simulink model "ref_controller"  (R2022b)
settings: Solver=VariableStepAuto  StartTime=0.0  StopTime=100.0  RelTol=1e-5
settings Model: Creator=marne  LastModifiedBy=marne

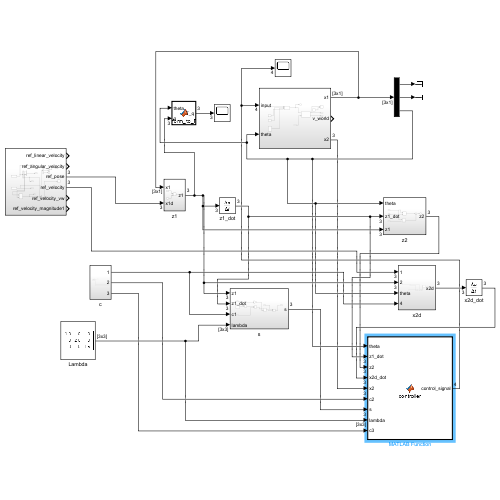
[thumbnail: Simulink's stored preview of the top-level diagram]
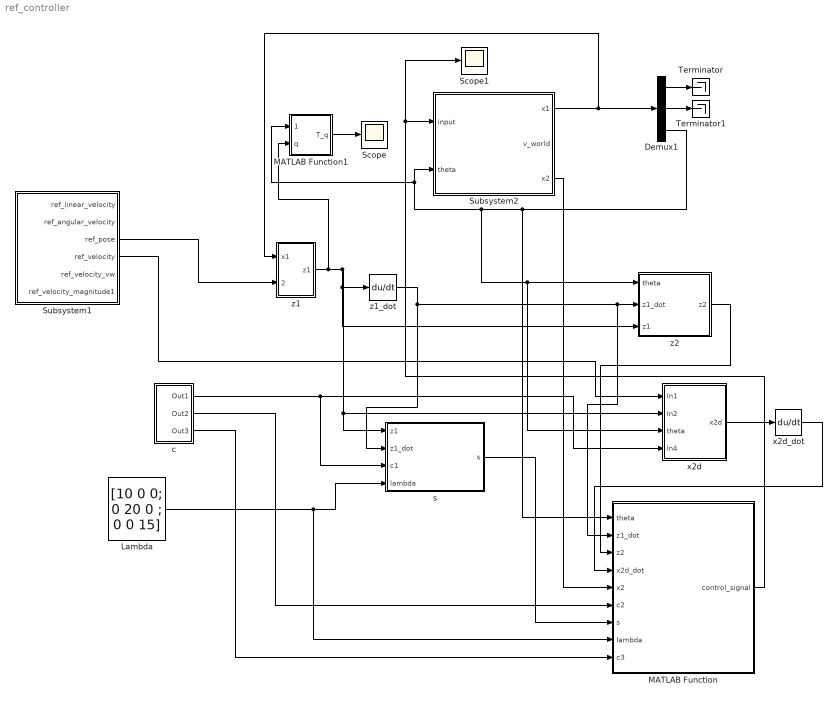
== system ref_controller ==
  Demux1 : Demux  Outputs=3
  Lambda : Constant  Value=[10 0 0; 0 20 0 ; 0 0 15]  VectorParams1D=off
  MATLAB Function : MATLAB Function  TreatAsAtomicUnit=on
  MATLAB Function1 : MATLAB Function  TreatAsAtomicUnit=on
  Scope : Scope
  Scope1 : Scope
  Subsystem1 : Subsystem
  Subsystem2 : Subsystem
  Terminator : Terminator
  Terminator1 : Terminator
  c : Subsystem
  s : Subsystem
  x2d : Subsystem
  x2d_dot : Derivative
  z1 : Subsystem
  z1_dot : Derivative
  z2 : Subsystem
  wires:
  Subsystem1/3(ref_pose) -> z1/2(x1d)
  Subsystem1/4(ref_velocity) -> x2d/1(In1)
  x2d/1(x2d) -> x2d_dot/1
  z1_dot/1 -> s/2(z1_dot), MATLAB Function/2(z1_dot), z2/2(z1_dot)
  z1/1(z1) -> MATLAB Function1/2(q), z2/3(z1), z1_dot/1, s/1(z1), x2d/2(In2)
  Lambda/1 -> MATLAB Function/8(lambda), s/4(lambda)
  Subsystem2/1(x1) -> z1/1(x1), Demux1/1
  Demux1/3 -> MATLAB Function/1(theta), x2d/3(theta), z2/1(theta), MATLAB Function1/1(theta), Subsystem2/2(theta)
  s/1(s) -> MATLAB Function/7(s)
  x2d_dot/1 -> MATLAB Function/4(x2d_dot)
  Subsystem2/3(x2) -> MATLAB Function/5(x2)
  z2/1(z2) -> MATLAB Function/3(z2)
  MATLAB Function/1(control_signal) -> Scope1/1, Subsystem2/1(input)
  Demux1/1 -> Terminator/1
  Demux1/2 -> Terminator1/1
  c/1(Out1) -> s/3(c1), x2d/4(In4)
  c/2(Out2) -> MATLAB Function/6(c2)
  c/3(Out3) -> MATLAB Function/9(c3)
  MATLAB Function1/1(T_q) -> Scope/1

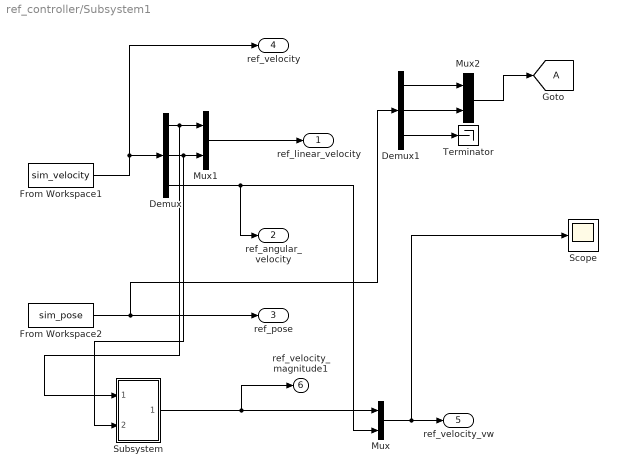
== system ref_controller/Subsystem1 ==
  Demux : Demux  Outputs=3
  Demux1 : Demux  Outputs=3
  From Workspace1 : FromWorkspace  VariableName=sim_velocity  OutputAfterFinalValue=Setting to zero
  From Workspace2 : FromWorkspace  VariableName=sim_pose  OutputAfterFinalValue=Setting to zero
  Goto : Goto  TagVisibility=global
  Mux : Mux  Inputs=2
  Mux1 : Mux  Inputs=2
  Mux2 : Mux  Inputs=2
  Scope : Scope
  Subsystem : Subsystem
  Terminator : Terminator
  ref_linear_velocity : Outport
  ref_angular_velocity : Outport  Port=2
  ref_pose : Outport  Port=3
  ref_velocity : Outport  Port=4
  ref_velocity_vw : Outport  Port=5
  ref_velocity_magnitude1 : Outport  Port=6
  wires:
  From Workspace1/1 -> ref_velocity/1, Demux/1
  From Workspace2/1 -> Demux1/1, ref_pose/1
  Demux/1 -> Subsystem/1(In1), Mux1/1
  Demux/2 -> Subsystem/2(In2), Mux1/2
  Mux/1 -> Scope/1, ref_velocity_vw/1
  Demux/3 -> ref_angular_velocity/1, Mux/2
  Mux1/1 -> ref_linear_velocity/1
  Subsystem/1(Out1) -> Mux/1, ref_velocity_magnitude1/1
  Demux1/1 -> Mux2/1
  Demux1/2 -> Mux2/2
  Mux2/1 -> Goto/1
  Demux1/3 -> Terminator/1

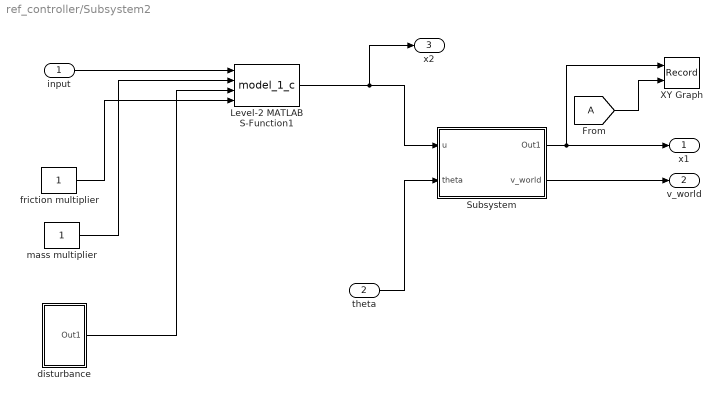
== system ref_controller/Subsystem2 ==
  input : Inport
  theta : Inport  Port=2
  From : From  TagVisibility=global
  Level-2 MATLAB S-Function1 : M-S-Function  FunctionName=model_1_c
  Subsystem : Subsystem
  XY Graph : Record  FileSettingsInternal="{\"entries\":[{\"content\":{\"excelSettings\":{\"content\":{},\"type\":\"Streamout.ExcelSettings\"}},\"type\":\"Streamout.FileSettingStorage\",\"uuid\":\"ee74998f-52cb-4860-92a7-c3e8b4709b8f\"}],\"packageUris\":[\"http://schema.mathworks.com/mf0/streamout_blocks/R2020a\"],\"version\":\"1.0\"}"  Layout=[1 1]  SignalsInternal="{\"entries\":[{\"content\":{\"signals\":[{\"content\":{\"blockPath\":[\"ref_controller/Subsystem2/XY Graph\"],\"channel\":[],\"dimensions\":[3,1],\"domain\":\"ref_controller/Subsystem2/XY Graph\",\"hasChildren\":true,\"lineColor\":\"#4dbeee\",\"plots\":[],\"port\":1,\"sid\":[\"\"],\"signalID\":23782,\"signalName\":\"Subsystem:1\"},\"type\":\"RecordBlkView.Signal\",\"uuid\":\"6d530b1b-06f5-4b68-9082-3b34886d0198\"},{\"content\":{\"blockPath\":[\"ref_controller/Subsystem2/XY Graph\"],\"channel\":[1,1],\"dimensions\":[3,1],\"domain\":\"ref_controller/Subsystem2/XY Graph\",\"lineColor\":\"#77ac30\",\"parentID\":23782,\"plots\":[1],\"port\":1,\"sid\":[\"\"],\"signalID\":23783,\"signalName\":\"Subsystem:1\"},\"type\":\"RecordBlkView.Signal\",\"uuid\":\"911fc2bd-e5fa-4a55-b3ae-83fe97ef8bd4\"},{\"content\":{\"blockPath\":[\"ref_controller/Subsystem2/XY Graph\"],\"channel\":[],\"dimensions\":[2],\"domain\":\"ref_controller/Subsystem2/XY Graph\",\"hasChildren\":true,\"lineColor\":\"#139fff\",\"plots\":[],\"port\":2,\"sid\":[\"\"],\"signalID\":23787,\"signalName\":\"From\"},\"type\":\"RecordBlkView.Signal\",\"uuid\":\"1cd1c2a0-0f57-43a7-b25a-7fd40aecd979\"},{\"content\":{\"blockPath\":[\"ref_controller/Subsystem2/XY Graph\"],\"channel\":[1],\"dimensions\":[2],\"domain\":\"ref_controller/Subsystem2/XY Graph\",\"lineColor\":\"#a2142f\",\"parentID\":23787,\"plots\":[1],\"port\":2,\"sid\":[\"\"],\"signalID\":23788,\"signalName\":\"From\"},\"type\":\"RecordBlkView.Signal\",\"uuid\":\"c857178d-09f4-4f1b-a9ee-64e8941ae8d6\"},{\"content\":{\"blockPath\":[\"ref_controller/Subsystem2/XY Graph\"],\"channel\":[2,1],\"dimensions\":[3,1],\"domain\":\"ref_controller/Subsystem2/XY Graph\",\"lineColor\":\"#139fff\",\"parentID\":23782,\"plots\":[1],\"port\":1,\"sid\":[\"\"],\"signalID\":23792,\"signalName\":\"Subsystem:1\"},\"type\":\"RecordBlkView.Signal\",\"uuid\":\"7d5dd58b-e2c6-4539-988b-1035a439ee67\"},{\"content\":{\"blockPath\":[\"ref_controller/Subsystem2/XY Graph\"],\"channel\":[3,1],\"dimensions\":[3,1],\"domain\":\"ref_controller/Subsystem2/XY Graph\",\"lineColor\":\"#ff6929\",\"parentID\":23782,\"plots\":[],\"port\":1,\"sid\":[\"\"],\"signalID\":23793,\"signalName\":\"Subsystem:1\"},\"type\":\"RecordBlkView.Signal\",\"uuid\":\"1922f216-f7cb-4e88-834d-1041113370d6\"},{\"content\":{\"blockPath\":[\"ref_controller/Subsystem2/XY Graph\"],\"channel\":[2],\"dimensions\":[2],\"domain\":\"ref_controller/Subsystem2/XY Graph\",\"lineColor\":\"#b746ff\",\"parentID\":23787,\"plots\":[1],\"port\":2,\"sid\":[\"\"],\"signalID\":23794,\"signalName\":\"From\"},\"type\":\"RecordBlkView.Signal\",\"uuid\":\"00801f00-9719-4b43-8906-470f49133c31\"}]},\"type\":\"RecordBlkView.InputSignals\",\"uuid\":\"772ae3a7-54e6-4943-ae8a-250a37e9e293\"}],\"packageUris\":[\"http://schema.mathworks.com/mf0/streamout_blocks/R2020a\"],\"version\":\"1.0\"}"  VisualizationBindings="{\"xyplotplugin\":{\"info\":[{\"series\":[{\"bindingParametersList\":[{\"parameter\":\"X-Axis\",\"signalID\":23783,\"signalName\":\"Subsystem:1(1,1)\"},{\"parameter\":\"Y-Axis\",\"signalID\":23792,\"signalName\":\"Subsystem:1(2,1)\"}],\"seriesID\":718},{\"bindingParametersList\":[{\"parameter\":\"X-Axis\",\"signalID\":23788,\"signalName\":\"From(1)\"},{\"parameter\":\"Y-Axis\",\"signalID\":23794,\"signalName\":\"From(2)\"}],\"seriesID\":954}],\"subplotID\":1}]}}"  CompatibilityTag=XY
  disturbance : Subsystem
  friction multiplier : Constant  VectorParams1D=off
  mass multiplier : Constant  VectorParams1D=off
  x1 : Outport
  v_world : Outport  Port=2
  x2 : Outport  Port=3
  wires:
  friction multiplier/1 -> Level-2 MATLAB S-Function1/4
  Subsystem/2(v_world) -> v_world/1
  mass multiplier/1 -> Level-2 MATLAB S-Function1/2
  Level-2 MATLAB S-Function1/1 -> x2/1, Subsystem/1(u)
  disturbance/1(Out1) -> Level-2 MATLAB S-Function1/3
  Subsystem/1(Out1) -> XY Graph/1, x1/1
  input/1 -> Level-2 MATLAB S-Function1/1
  theta/1 -> Subsystem/2(theta)
  From/1 -> XY Graph/2

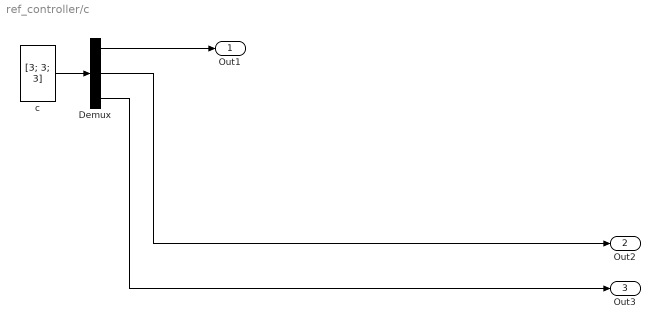
== system ref_controller/c ==
  Demux : Demux  Outputs=3
  c : Constant  Value=[3; 3; 3]  VectorParams1D=off
  Out1 : Outport
  Out2 : Outport  Port=2
  Out3 : Outport  Port=3
  wires:
  c/1 -> Demux/1
  Demux/1 -> Out1/1
  Demux/2 -> Out2/1
  Demux/3 -> Out3/1

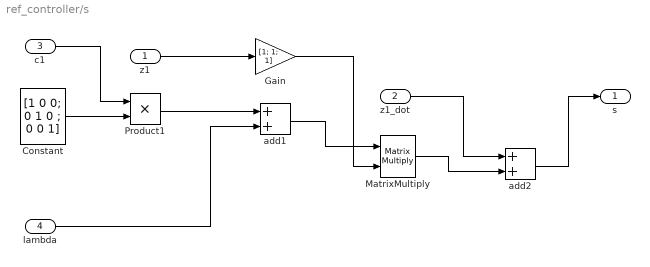
== system ref_controller/s ==
  z1 : Inport
  z1_dot : Inport  Port=2
  c1 : Inport  Port=3
  lambda : Inport  Port=4
  Constant : Constant  Value=[1 0 0; 0 1 0 ; 0 0 1]  VectorParams1D=off
  Gain : Gain  Gain=[1; 1; 1]
  MatrixMultiply : Product  Multiplication=Matrix(*)
  Product1 : Product
  add1 : Sum
  add2 : Sum
  s : Outport
  wires:
  add2/1 -> s/1
  c1/1 -> Product1/1
  z1/1 -> Gain/1
  z1_dot/1 -> add2/1
  lambda/1 -> add1/2
  add1/1 -> MatrixMultiply/1
  Constant/1 -> Product1/2
  Product1/1 -> add1/1
  Gain/1 -> MatrixMultiply/2
  MatrixMultiply/1 -> add2/2

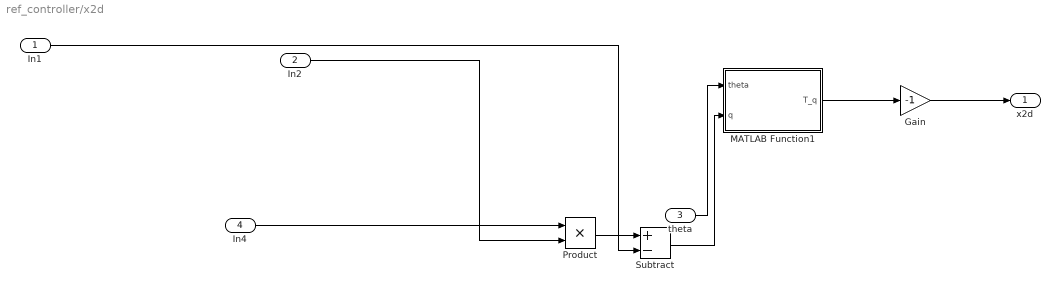
== system ref_controller/x2d ==
  In1 : Inport
  In2 : Inport  Port=2
  theta : Inport  Port=3
  In4 : Inport  Port=4
  Gain : Gain  Gain=-1
  MATLAB Function1 : MATLAB Function  TreatAsAtomicUnit=on
  Product : Product
  Subtract : Sum  Inputs=+-
  x2d : Outport
  wires:
  In1/1 -> Subtract/2
  In2/1 -> Product/2
  Subtract/1 -> MATLAB Function1/2(q)
  Product/1 -> Subtract/1
  theta/1 -> MATLAB Function1/1(theta)
  In4/1 -> Product/1
  MATLAB Function1/1(T_q) -> Gain/1
  Gain/1 -> x2d/1

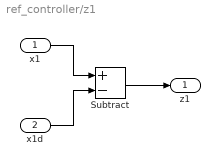
== system ref_controller/z1 ==
  x1 : Inport
  x1d : Inport  Port=2
  Subtract : Sum  Inputs=+-
  z1 : Outport
  wires:
  Subtract/1 -> z1/1
  x1/1 -> Subtract/1
  x1d/1 -> Subtract/2

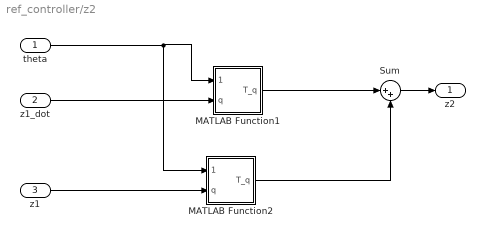
== system ref_controller/z2 ==
  theta : Inport
  z1_dot : Inport  Port=2
  z1 : Inport  Port=3
  MATLAB Function1 : MATLAB Function  TreatAsAtomicUnit=on
  MATLAB Function2 : MATLAB Function  TreatAsAtomicUnit=on
  Sum : Sum  Inputs=|++
  z2 : Outport
  wires:
  theta/1 -> MATLAB Function1/1(theta), MATLAB Function2/1(theta)
  MATLAB Function2/1(T_q) -> Sum/2
  MATLAB Function1/1(T_q) -> Sum/1
  z1_dot/1 -> MATLAB Function1/2(q)
  z1/1 -> MATLAB Function2/2(q)
  Sum/1 -> z2/1

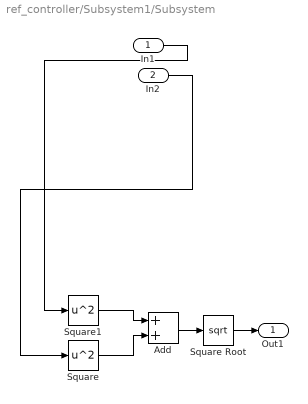
== system ref_controller/Subsystem1/Subsystem ==
  In1 : Inport
  In2 : Inport  Port=2
  Add : Sum
  Square : Math  Operator=square
  Square Root : Sqrt
  Square1 : Math  Operator=square
  Out1 : Outport
  wires:
  Add/1 -> Square Root/1
  Square1/1 -> Add/1
  In2/1 -> Square/1
  Square/1 -> Add/2
  Square Root/1 -> Out1/1
  In1/1 -> Square1/1

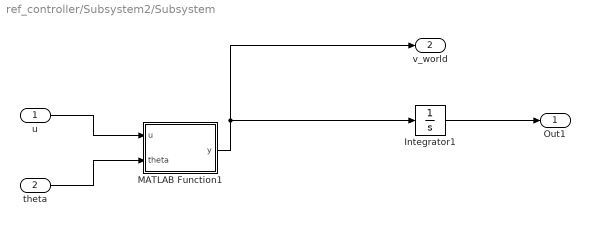
== system ref_controller/Subsystem2/Subsystem ==
  u : Inport
  theta : Inport  Port=2
  Integrator1 : Integrator  InitialCondition=[0;0;0]
  MATLAB Function1 : MATLAB Function  TreatAsAtomicUnit=on
  Out1 : Outport
  v_world : Outport  Port=2
  wires:
  Integrator1/1 -> Out1/1
  u/1 -> MATLAB Function1/1(u)
  theta/1 -> MATLAB Function1/2(theta)
  MATLAB Function1/1(y) -> v_world/1, Integrator1/1

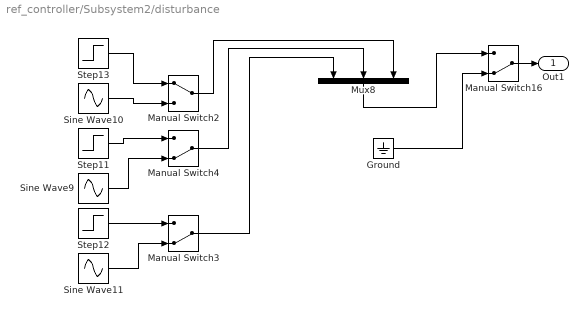
== system ref_controller/Subsystem2/disturbance ==
  Ground : Ground
  Manual Switch16 : ManualSwitch  CurrentSetting=0
  Manual Switch2 : ManualSwitch
  Manual Switch3 : ManualSwitch  CurrentSetting=0
  Manual Switch4 : ManualSwitch  CurrentSetting=0
  Mux8 : Mux  Inputs=3
  Sine Wave10 : Sin  Amplitude=2  Frequency=2  Phase=3  SampleTime=0
  Sine Wave11 : Sin  Frequency=2  Phase=1  SampleTime=0
  Sine Wave9 : Sin  Frequency=2  Phase=2  SampleTime=0
  Step11 : Step  Time=8  SampleTime=0
  Step12 : Step  Time=5  SampleTime=0
  Step13 : Step  Time=13  SampleTime=0
  Out1 : Outport
  wires:
  Step13/1 -> Manual Switch2/1
  Manual Switch3/1 -> Mux8/1
  Sine Wave11/1 -> Manual Switch3/2
  Mux8/1 -> Manual Switch16/1
  Sine Wave10/1 -> Manual Switch2/2
  Step11/1 -> Manual Switch4/1
  Step12/1 -> Manual Switch3/1
  Sine Wave9/1 -> Manual Switch4/2
  Manual Switch2/1 -> Mux8/3
  Ground/1 -> Manual Switch16/2
  Manual Switch4/1 -> Mux8/2
  Manual Switch16/1 -> Out1/1

== matlab function ref_controller/MATLAB Function1 ==
  data: theta input; T_q output; q input
function T_q = Transform_to_Robot(theta,q)


q_robot_rotation = [cos(theta) sin(theta) 0
                   -sin(theta) cos(theta) 0
                      0           0       1];
        
T_q = q_robot_rotation * q;

== matlab function ref_controller/z2/MATLAB Function1 ==
  data: theta input; T_q output; q input
function T_q = Transform_to_Robot(theta,q)


q_robot_rotation = [cos(theta) sin(theta) 0
                   -sin(theta) cos(theta) 0
                      0           0       1];
        
T_q = q_robot_rotation * q;

== matlab function ref_controller/z2/MATLAB Function2 ==
  data: theta input; T_q output; q input
function T_q = Transform_to_Robot(theta,q)


q_robot_rotation = [cos(theta) sin(theta) 0
                   -sin(theta) cos(theta) 0
                      0           0       1];
        
T_q = q_robot_rotation * q;

== matlab function ref_controller/x2d/MATLAB Function1 ==
  data: theta input; T_q output; q input
function T_q = Transform_to_Robot(theta,q)


q_robot_rotation = [cos(theta) sin(theta) 0
                   -sin(theta) cos(theta) 0
                      0           0       1];
        
T_q = q_robot_rotation * q;

== matlab function ref_controller/MATLAB Function ==
  data: theta input; control_signal output; z1_dot input; z2 input; x2d_dot input; x2 input; c2 input; s input; lambda input; c3 input
function control_signal = controller(theta,z1_dot,z2,x2d_dot,x2,c2,s,lambda,c3)
%function control_signal = controller(theta,z1_dot,z2,x2d_dot,x2,c2,s,c3)
persistent flag;

 
    %lambda = blkdiag(10,20,15);


Bpinv =  [     0    0.3628    0.0217
   -0.2857   -0.0000    0.0276
         0   -0.3628    0.0217
    0.2857    0.0000    0.0276];

C = [78.7605         0         0
         0   49.8330         0
         0         0    5.5910];

M = [ 35   0     0
     0    35     0
     0     0     1.37];

H_inv = [cos(theta) sin(theta) 0
        -sin(theta) cos(theta) 0 
           0           0       1];


H_dot = [-sin(theta) -cos(theta) 0
          cos(theta) -sin(theta) 0
          0             0        0];


G  =  [29.4490         0     0
         0   29.6100         0
         0         0    5.1200];

control_signal = -Bpinv*(M*(H_inv*(lambda*z1_dot+H_dot*z2)-x2d_dot)-C*x2-G*tanh(10*x2))-...
    Bpinv*M*H_inv*(c2*eye(3)*tanh(10*s)+c3*eye(3)*s);

== matlab function ref_controller/Subsystem2/Subsystem/MATLAB Function1 ==
  data: u input; y output; theta input
function y = Rot(u,theta)
y = [ cos(theta) -sin(theta) 0; 
      sin(theta) cos(theta) 0;
       0 0 1] * u;
